simulink model "model"  (R2017b)
settings: Solver=ode4  StartTime=0.0  StopTime=10.0  FixedStep=2^-7  RelTol=1e-3
libraries: simulink x2
settings Model: Creator=mt35448  LastModifiedBy=mt35448

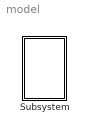
== system model ==
  Subsystem : Subsystem  mask{M=100, G=9.81, R=2, vx0=10, vy0=0, Rs=0.02, x0=0, y0=5}
      mask prompts: vx0 "Vx(0)"; vy0 "Vy(0)"

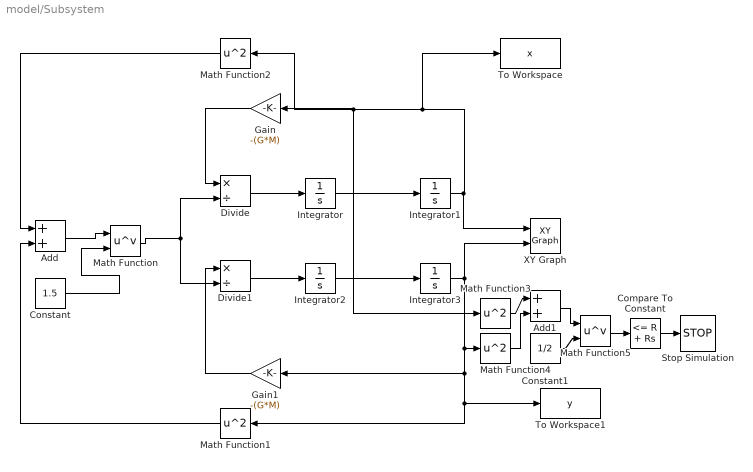
== system model/Subsystem ==
  Add : Sum
  Add1 : Sum
  Compare To Constant : simulink/Logic and Bit Operations/Compare To Constant  relop=<=  const=R + Rs  OutDataTypeStr=boolean
  Constant : Constant  Value=1.5
  Constant1 : Constant  Value=1/2
  Divide : Product  Inputs=*/
  Divide1 : Product  Inputs=*/
  Gain : Gain  Gain=-(G*M)
  Gain1 : Gain  Gain=-(G*M)
  Integrator : Integrator  InitialCondition=vx0
  Integrator1 : Integrator  InitialCondition=x0
  Integrator2 : Integrator  InitialCondition=vy0
  Integrator3 : Integrator  InitialCondition=y0
  Math Function : Math  Operator=pow  SaturateOnIntegerOverflow=on
  Math Function{1..4} (4 alike) : Math  Operator=square  SaturateOnIntegerOverflow=on
  Math Function5 : Math  Operator=pow  SaturateOnIntegerOverflow=on
  Stop Simulation : Stop
  To Workspace : ToWorkspace  VariableName=x  SampleTime=-1
      settings: Save2DSignal=2-D array (concatenate along first dimension)
  To Workspace1 : ToWorkspace  VariableName=y  SampleTime=-1
      settings: Save2DSignal=2-D array (concatenate along first dimension)
  XY Graph : simulink/Sinks/XY Graph  xmin=-10  xmax=10  ymin=-10  ymax=10  st=-1
  wires:
  Add/1 -> Math Function/1
  Integrator1/1 -> XY Graph/1, To Workspace/1, Math Function2/1, Gain/1, Math Function3/1
  Gain/1 -> Divide/1
  Math Function2/1 -> Add/1
  Math Function1/1 -> Add/2
  Integrator3/1 -> XY Graph/2, Gain1/1, To Workspace1/1, Math Function1/1, Math Function4/1
  Math Function/1 -> Divide1/2, Divide/2
  Constant/1 -> Math Function/2
  Gain1/1 -> Divide1/1
  Divide/1 -> Integrator/1
  Integrator2/1 -> Integrator3/1
  Divide1/1 -> Integrator2/1
  Integrator/1 -> Integrator1/1
  Compare To Constant/1 -> Stop Simulation/1
  Add1/1 -> Math Function5/1
  Math Function3/1 -> Add1/1
  Math Function4/1 -> Add1/2
  Constant1/1 -> Math Function5/2
  Math Function5/1 -> Compare To Constant/1
